simulink model "Motor_controller"  (R2024b)
settings: Solver=VariableStepAuto  StartTime=0.0  StopTime=10.0  RelTol=1e-3
values from neighbouring files (symbols this model uses):
  a = -21212/c    (= -13.249219238)    [Controller.m]    (also in Controller2.m; Controller_motor_only.m = -15.4812967581; motor_control.m)
  b = 21104/c    (= 13.1817613991)    [Controller.m]    (also in Controller2.m; Controller_motor_only.m = 15.421446384; motor_control.m)
  d = -1599/c    (= -0.998750780762)    [Controller.m]    (also in Controller2.m; Controller_motor_only.m = 0.995012468828; motor_control.m)
  Ts = 0.01    [Controller.m]    (also in Controller2.m; Controller_motor_only.m; State_Space_Controller.m; dist_translate.m)
libraries: simulink x1, cstblocks x1
settings Model: Creator=ethan  LastModifiedBy=ethan

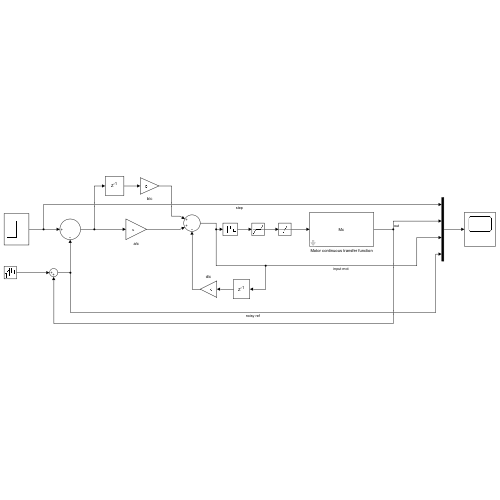
[thumbnail: Simulink's stored preview of the top-level diagram]
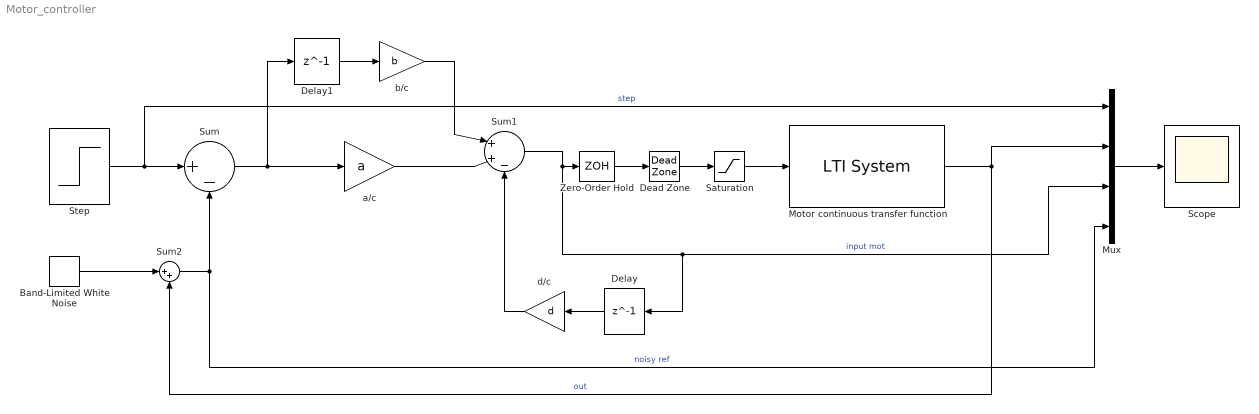
== system Motor_controller ==
  Band-Limited White Noise : simulink/Sources/Band-Limited White Noise  Cov=[0.00005]  Ts=Ts  seed=[23341]
  Dead Zone : DeadZone  LowerValue=-1.75  UpperValue=1.7
  Delay : Delay  DelayLength=1  InputProcessing=Columns as channels (frame based)
  Delay1 : Delay  DelayLength=1  InputProcessing=Columns as channels (frame based)
  Motor continuous transfer function : cstblocks/LTI System  sys=Mc  IC=[]  PadeOrder=0
  Mux : Mux
  Saturation : Saturate  UpperLimit=8.30  LowerLimit=-8.42
  Scope : Scope
  Step : Step  SampleTime=0
  Sum : Sum  Inputs=|+-
  Sum1 : Sum  Inputs=|++-
  Sum2 : Sum  Inputs=|++
  Zero-Order Hold : ZeroOrderHold  SampleTime=0.01
  a/c : Gain  Gain=a
  b/c : Gain  Gain=b
  d/c : Gain  Gain=d
  wires:
  Step/1 -> Sum/1, Mux/1  "step"
  Motor continuous transfer function/1 -> Sum2/2, Mux/2  "out"
  Sum/1 -> a/c/1, Delay1/1
  Delay1/1 -> b/c/1
  a/c/1 -> Sum1/2
  b/c/1 -> Sum1/1
  Delay/1 -> d/c/1
  d/c/1 -> Sum1/3
  Sum1/1 -> Zero-Order Hold/1, Delay/1, Mux/3  "input mot"
  Mux/1 -> Scope/1
  Zero-Order Hold/1 -> Dead Zone/1
  Saturation/1 -> Motor continuous transfer function/1
  Dead Zone/1 -> Saturation/1
  Band-Limited White Noise/1 -> Sum2/1
  Sum2/1 -> Sum/2, Mux/4  "noisy ref"
